simulink model "q8_sem_deadzone"  (R2025b)
settings: Solver=VariableStepAuto  StartTime=0.0  StopTime=20  RelTol=1e-3
values from neighbouring files (symbols this model uses):
  A = [0 0 0 0 0 1 -0.0174048595758 0 -0.0173759205618 -232.025201375 0 20.7861247087 ... (25 elements, 5x5)]    [teste_03_03_26.mat]
  B = [0 0 0 0 333.33674813]    [teste_03_03_26.mat]
  C = eye(5)    [q6.m]    (also in teste_03_03_26.mat = [1  0  0  0  0; 0  0  1  0  0])
  D = [0 0 0 0 0]'    [q6.m]    (also in teste_03_03_26.mat = [0 0])
  D_estim = zeros(1,2)    [q8.m]
  estim_A = A - B*K - L*C    [q8.m]
  K = lqr(A, B, Qr, Rr)    [q6.m]    (also in teste_03_03_26.mat = [-9.99999999994 -4.90890463799 39.8345312888 5.91812225181 0)
  L = lqe(A, G, C, Qe, Re)    [q7.m]    (also in q8.m; teste_03_03_26.mat = [3.26664981927  1.13709483629; 0.981992854244  11.8725297148)
  x0 = [0.1 0 0 0 0]'    [q6.m]    (also in q8.m)
settings Model: Creator=matos  LastModifiedBy=matos

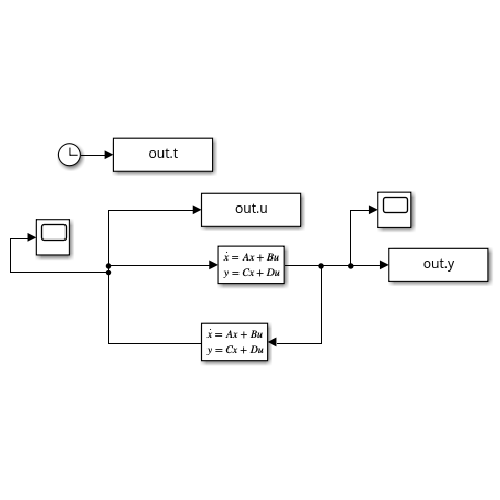
[thumbnail: Simulink's stored preview of the top-level diagram]
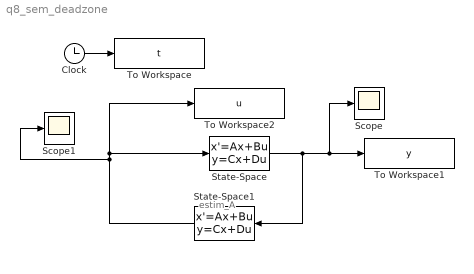
== system q8_sem_deadzone ==
  note: estim_A
  Clock : Clock
  Scope : Scope
      settings: ActiveDisplayYMinimum=-0.018324001872298344  ActiveDisplayYMaximum=0.12112647393831649
  Scope1 : Scope
  State-Space : StateSpace  A=A  B=B  C=C  D=D  InitialCondition=x0
  State-Space1 : StateSpace  A=estim_A  B=L  C=-K  D=D_estim  InitialCondition=0
  To Workspace : ToWorkspace  VariableName=t  SaveFormat=Timeseries  SampleTime=-1
  To Workspace1 : ToWorkspace  VariableName=y  SaveFormat=Timeseries  SampleTime=-1
  To Workspace2 : ToWorkspace  VariableName=u  SaveFormat=Timeseries  SampleTime=-1
  wires:
  Clock/1 -> To Workspace/1
  State-Space/1 -> Scope/1, To Workspace1/1, State-Space1/1
  State-Space1/1 -> Scope1/1, State-Space/1, To Workspace2/1
